simulink model "Position_Controller_V2"  (Simulink 8.9)
settings: Solver=ode45  StartTime=0.0  StopTime=1  RelTol=1e-3
settings Model: Creator=MONSTER  LastModifiedBy=MONSTER
settings SolverCC: ZeroCrossAlgorithm=Adaptive
settings DataIOCC: LimitDataPoints=off  SaveFormat=Dataset  SignalLoggingSaveFormat=Dataset
settings OptimizationCC: LifeSpan=auto
settings DebuggingCC: UnderspecifiedInitializationDetection=Simplified  MergeDetectMultiDrivingBlocksExec=error  FcnCallInpInsideContextMsg=error  StateNameClashWarn=none  SFUnexpectedBacktrackingDiag=error  SFNoUnconditionalDefaultTransitionDiag=error  SFExecutionAtInitializationDiag=warning
settings HardwareCC: ProdBitPerPointer=64  ProdBitPerSizeT=64  ProdBitPerPtrDiffT=64  ProdLargestAtomicFloat=Float  ProdIntDivRoundTo=Zero  ProdEndianess=LittleEndian  ProdWordSize=64  ProdHWDeviceType=Intel->x86-64 (Windows64)
settings ModelReferenceCC: PropagateSignalLabelsOutOfModel=on
settings GRTTargetCC: TargetLangStandard=C99 (ISO)  GeneratePreprocessorConditionals=Use local settings  CombineOutputUpdateFcns=on  GRTInterface=off
settings ConfigComp: CovMetricSettings=dwe  CovHtmlReporting=off  CovSaveCumulativeToWorkspaceVar=off  CovSaveSingleToWorkspaceVar=off  CovExternalEMLEnable=on

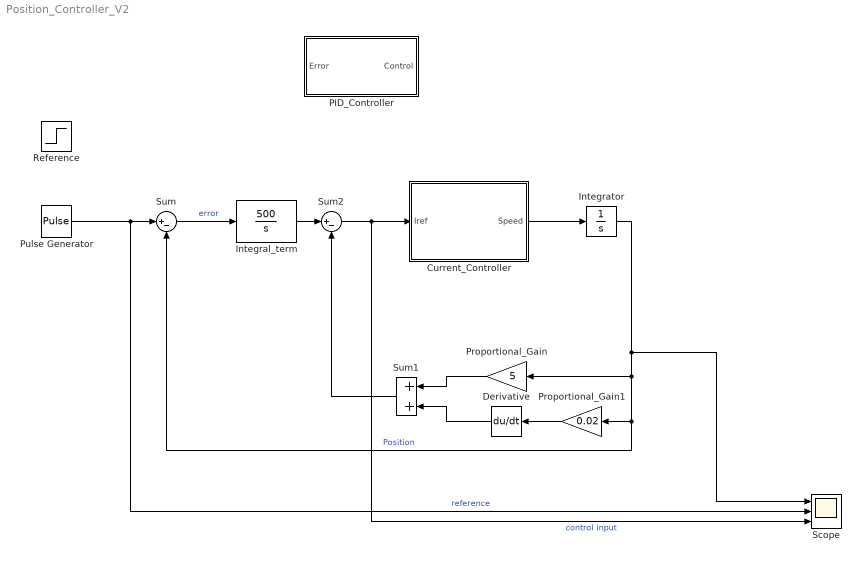
== system Position_Controller_V2 ==
  "Current_Controller " : Subsystem
  Derivative : Derivative
  "Integral_term " : TransferFcn  Numerator=500  Denominator=[1 0]
  Integrator : Integrator
  PID_Controller : Subsystem
  Proportional_Gain : Gain  Gain=5
  Proportional_Gain1 : Gain  Gain=0.02
  Pulse Generator : DiscretePulseGenerator  PulseType=Time based  Amplitude=3.14  Period=0.2  PulseWidth=50
  Reference : Step  Time=0.1  After=1.6  SampleTime=0
  Scope : Scope  NumInputPorts=3
  Sum : Sum  Inputs=|+-
  Sum1 : Sum
  Sum2 : Sum  Inputs=|+-
  wires:
  Pulse Generator/1 -> Scope/2, Sum/1  "reference"
  Sum2/1 -> Scope/3, "Current_Controller "/1(Iref)  "control input"
  Sum/1 -> "Integral_term "/1  "error"
  "Current_Controller "/1(Speed) -> Integrator/1
  Sum1/1 -> Sum2/2
  Proportional_Gain/1 -> Sum1/1
  Integrator/1 -> Scope/1, Proportional_Gain/1, Proportional_Gain1/1, Sum/2  "Position"
  Derivative/1 -> Sum1/2
  Proportional_Gain1/1 -> Derivative/1
  "Integral_term "/1 -> Sum2/1

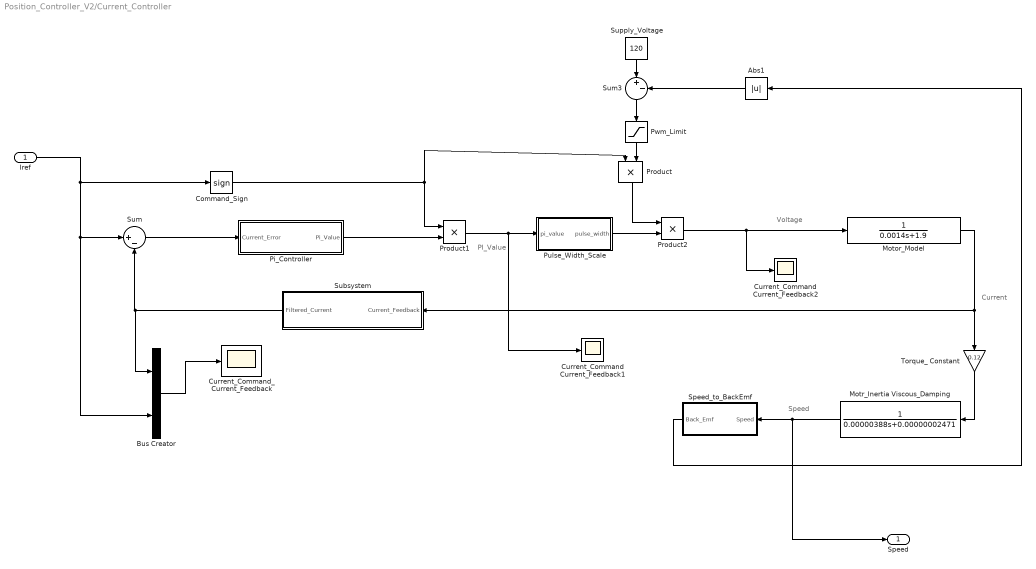
== system Position_Controller_V2/Current_Controller  ==
  note: Speed
  note: Current
  note: Voltage
  note: PI_Value
  Iref : Inport
  Abs1 : Abs
  Bus Creator : BusCreator  Inputs=2
  Command_Sign : Signum
  Current_Command Current_Feedback1 : Scope
  Current_Command Current_Feedback2 : Scope
  "Current_Command_ Current_Feedback " : Scope
  Motor_Model : TransferFcn  Denominator=[0.0014 1.9]
  Motr_Inertia Viscous_Damping : TransferFcn  Denominator=[0.00000388 0.00000002471]
  Pi_Controller : Subsystem
  Product : Product
  Product1 : Product
  Product2 : Product
  Pulse_Width_Scale : Subsystem
  Pwm_Limit : Saturate  UpperLimit=120  LowerLimit=0
  Speed_to_BackEmf : Subsystem
  Subsystem : Subsystem
  Sum : Sum  Inputs=|+-
  Sum3 : Sum  Inputs=|+-
  Supply_Voltage : Constant  Value=120
  Torque_ Constant : Gain  Gain=0.12
  Speed : Outport
  wires:
  Sum3/1 -> Pwm_Limit/1
  Product/1 -> Product2/1
  Supply_Voltage/1 -> Sum3/1
  Sum/1 -> Pi_Controller/1("Current_Error ")
  Pwm_Limit/1 -> Product/2
  Abs1/1 -> Sum3/2
  Product1/1 -> Current_Command Current_Feedback1/1, Pulse_Width_Scale/1(pi_value)
  Torque_ Constant/1 -> Motr_Inertia Viscous_Damping/1
  Subsystem/1("Filtered_Current ") -> Bus Creator/1, Sum/2
  Pulse_Width_Scale/1(pulse_width) -> Product2/2
  Command_Sign/1 -> Product1/1, Product/1
  Product2/1 -> Current_Command Current_Feedback2/1, Motor_Model/1
  Motor_Model/1 -> Subsystem/1(Current_Feedback), Torque_ Constant/1
  Bus Creator/1 -> "Current_Command_ Current_Feedback "/1
  Pi_Controller/1("Pi_Value ") -> Product1/2
  Motr_Inertia Viscous_Damping/1 -> Speed/1, Speed_to_BackEmf/1(Speed)
  Speed_to_BackEmf/1(Back_Emf) -> Abs1/1
  Iref/1 -> Command_Sign/1, Sum/1, Bus Creator/2

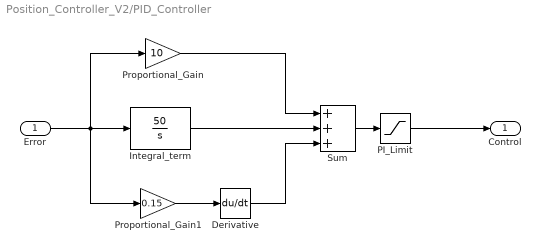
== system Position_Controller_V2/PID_Controller ==
  Error : Inport
  Derivative : Derivative
  "Integral_term " : TransferFcn  Numerator=50  Denominator=[1 0]
  PI_Limit : Saturate  UpperLimit=10  LowerLimit=-10
  Proportional_Gain : Gain  Gain=10
  Proportional_Gain1 : Gain  Gain=0.15
  Sum : Sum  Inputs=+++
  Control : Outport
  wires:
  PI_Limit/1 -> Control/1
  Proportional_Gain/1 -> Sum/1
  "Integral_term "/1 -> Sum/2
  Derivative/1 -> Sum/3
  Sum/1 -> PI_Limit/1
  Proportional_Gain1/1 -> Derivative/1
  Error/1 -> Proportional_Gain/1, "Integral_term "/1, Proportional_Gain1/1

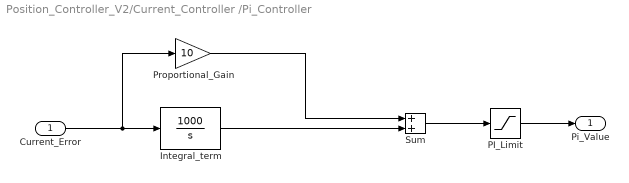
== system Position_Controller_V2/Current_Controller /Pi_Controller ==
  "Current_Error " : Inport
  "Integral_term " : TransferFcn  Numerator=1000  Denominator=[1 0]
  PI_Limit : Saturate  UpperLimit=10  LowerLimit=-10
  Proportional_Gain : Gain  Gain=10
  Sum : Sum
  "Pi_Value " : Outport
  wires:
  PI_Limit/1 -> "Pi_Value "/1
  Sum/1 -> PI_Limit/1
  Proportional_Gain/1 -> Sum/1
  "Integral_term "/1 -> Sum/2
  "Current_Error "/1 -> Proportional_Gain/1, "Integral_term "/1

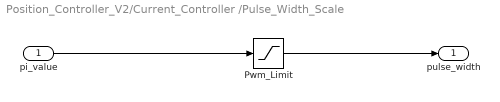
== system Position_Controller_V2/Current_Controller /Pulse_Width_Scale ==
  pi_value : Inport
  Pwm_Limit : Saturate  UpperLimit=1  LowerLimit=-1
  pulse_width : Outport
  wires:
  Pwm_Limit/1 -> pulse_width/1
  pi_value/1 -> Pwm_Limit/1

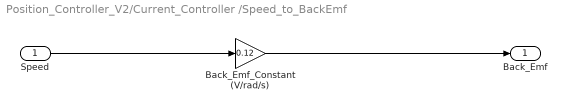
== system Position_Controller_V2/Current_Controller /Speed_to_BackEmf ==
  Speed : Inport
  Back_Emf_Constant (V/rad/s) : Gain  Gain=0.12
  Back_Emf : Outport
  wires:
  Speed/1 -> Back_Emf_Constant (V/rad/s)/1
  Back_Emf_Constant (V/rad/s)/1 -> Back_Emf/1

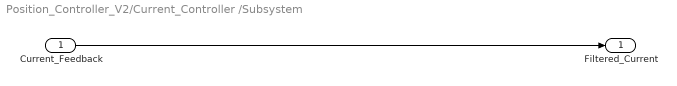
== system Position_Controller_V2/Current_Controller /Subsystem ==
  Current_Feedback : Inport
  "Filtered_Current " : Outport
  wires:
  Current_Feedback/1 -> "Filtered_Current "/1
